simulink model "recti_response"  (Simulink 9.1)
settings: Solver=ode4  StartTime=0.0  StopTime=10  FixedStep=0.001  RelTol=1e-3
settings Model: Creator=HuuNgan  LastModifiedBy=HuuNgan
settings DataIOCC: SaveFormat=Dataset
settings OptimizationCC: LifeSpan=auto
settings DebuggingCC: UnderspecifiedInitializationDetection=Simplified  MergeDetectMultiDrivingBlocksExec=error  SFUnexpectedBacktrackingDiag=error  SFNoUnconditionalDefaultTransitionDiag=error  SFExecutionAtInitializationDiag=warning
settings HardwareCC: ProdBitPerPointer=64  ProdBitPerSizeT=64  ProdBitPerPtrDiffT=64  ProdLargestAtomicFloat=Float  ProdIntDivRoundTo=Zero  ProdEndianess=LittleEndian  ProdWordSize=64  ProdHWDeviceType=Intel->x86-64 (Windows64)
settings ModelReferenceCC: PropagateSignalLabelsOutOfModel=on
settings CodeAppCC: StateflowObjectComments=off
settings GRTTargetCC: TargetLangStandard=C99 (ISO)  CombineOutputUpdateFcns=on  GRTInterface=off
settings ConfigComp: CovMetricSettings=dwe  CovHtmlReporting=off  CovSaveCumulativeToWorkspaceVar=off  CovSaveSingleToWorkspaceVar=off  CovExternalEMLEnable=on

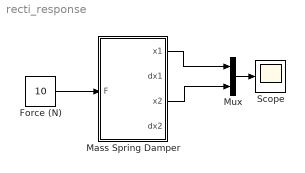
== system recti_response ==
  Force (N) : Constant  Value=10  SampleTime=0.001
  Mass Spring Damper : Subsystem
  Mux : Mux  Inputs=2
  "Scope " : Scope
  wires:
  Mux/1 -> "Scope "/1
  Mass Spring Damper/1(x1) -> Mux/1
  Mass Spring Damper/3(x2) -> Mux/2
  Force (N)/1 -> Mass Spring Damper/1(F)

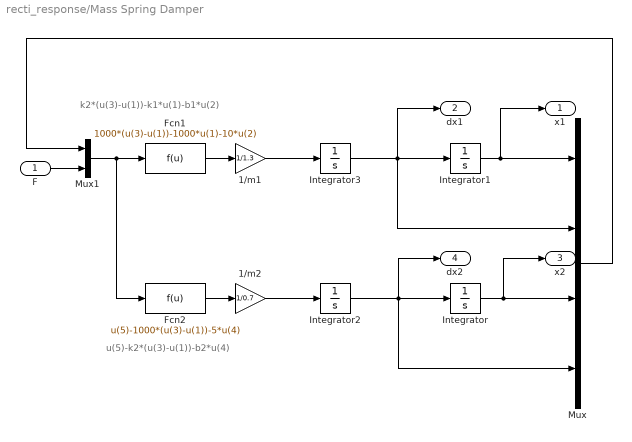
== system recti_response/Mass Spring Damper ==
  note: u(5)-k2*(u(3)-u(1))-b2*u(4)
  note: k2*(u(3)-u(1))-k1*u(1)-b1*u(2)
  F : Inport
  1/m1 : Gain  Gain=1/1.3
  1/m2 : Gain  Gain=1/0.7
  "Fcn1 " : Fcn  Expr=1000*(u(3)-u(1))-1000*u(1)-10*u(2)
  "Fcn2 " : Fcn  Expr=u(5)-1000*(u(3)-u(1))-5*u(4)
  Integrator{,1..3} (4 alike) : Integrator
  Mux : Mux
  Mux1 : Mux  Inputs=2
  x1 : Outport
  dx1 : Outport  Port=2
  x2 : Outport  Port=3
  dx2 : Outport  Port=4
  wires:
  1/m2/1 -> Integrator2/1
  "Fcn2 "/1 -> 1/m2/1
  F/1 -> Mux1/2
  Integrator/1 -> x2/1, Mux/3
  1/m1/1 -> Integrator3/1
  Mux1/1 -> "Fcn2 "/1, "Fcn1 "/1
  Integrator3/1 -> dx1/1, Mux/2, Integrator1/1
  Integrator2/1 -> dx2/1, Mux/4, Integrator/1
  Mux/1 -> Mux1/1
  "Fcn1 "/1 -> 1/m1/1
  Integrator1/1 -> x1/1, Mux/1
